simulink model "inverter"  (R2020b)
settings: Solver=VariableStepAuto  StartTime=0.0  StopTime=10.0  RelTol=1e-3
settings Model: Creator=omkar  LastModifiedBy=DELL

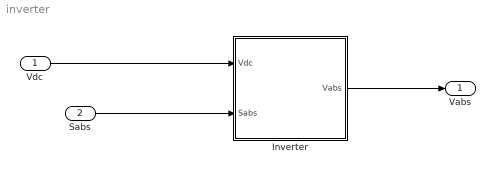
== system inverter ==
  Vdc : Inport
  Sabs : Inport  Port=2
  Inverter : Subsystem
  Vabs : Outport
  wires:
  Vdc/1 -> Inverter/1(Vdc)
  Sabs/1 -> Inverter/2(Sabs)
  Inverter/1(Vabs) -> Vabs/1

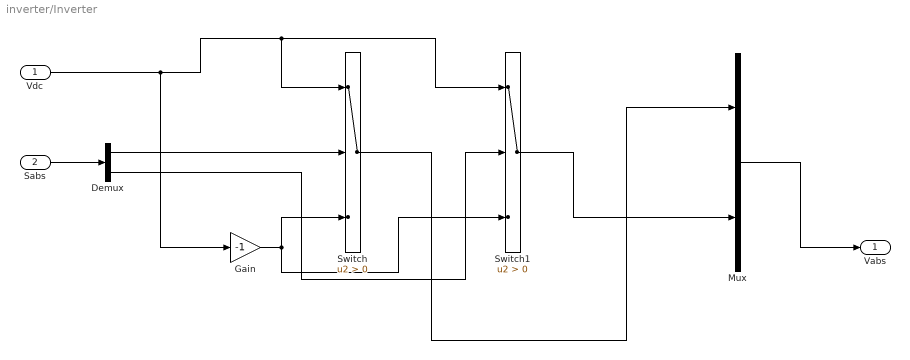
== system inverter/Inverter ==
  Vdc : Inport
  Sabs : Inport  Port=2
  Demux : Demux  Outputs=2
  Gain : Gain  Gain=-1
  Mux : Mux  Inputs=2
  Switch : Switch  Criteria=u2 > Threshold
  Switch1 : Switch  Criteria=u2 > Threshold
  Vabs : Outport
  wires:
  Demux/1 -> Switch/2
  Vdc/1 -> Gain/1, Switch/1, Switch1/1
  Gain/1 -> Switch/3, Switch1/3
  Mux/1 -> Vabs/1
  Switch1/1 -> Mux/2
  Demux/2 -> Switch1/2
  Switch/1 -> Mux/1
  Sabs/1 -> Demux/1
